simulink model "BenchmarkModel_Dynamic_TestCase"  (R2020a)
settings: Solver=ode45  StartTime=0.0  StopTime=5  RelTol=1e-3
undefined symbols (not defined in the file): Angle, D1, Delta, find_system, Magnitude
libraries: powerlib x91, powerlib_meascontrol x31, simulink x6, dspsrcs4 x3, dspsigops x2, sps_avr x1
(part 1 of 3)
settings Model: Creator=user  LastModifiedBy=anton

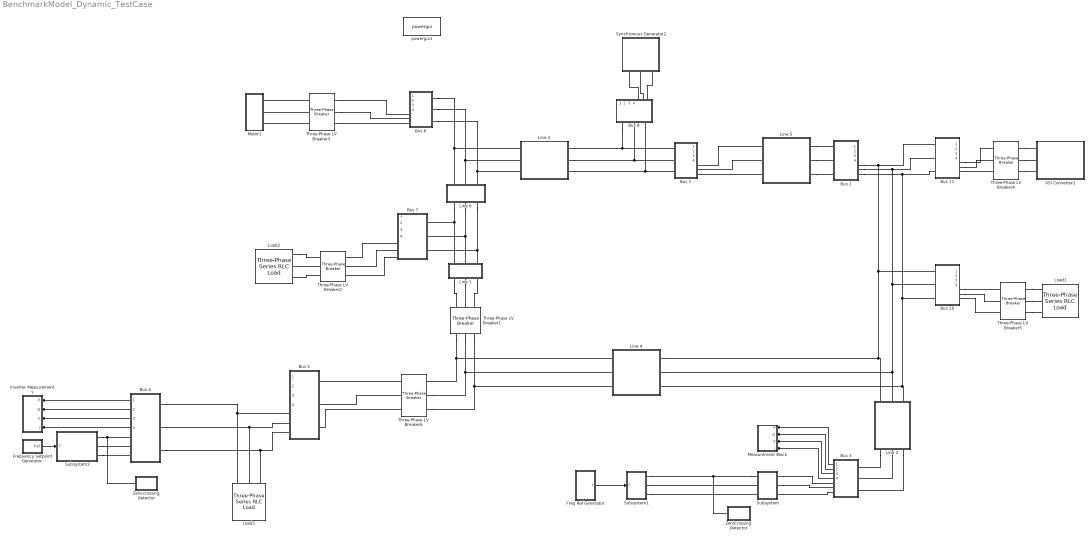
== system BenchmarkModel_Dynamic_TestCase ==
  Bus {1..8,10..11} (10 alike) : Subsystem  ReferencedSubsystem=Bus
  Freq Ref Generator : Subsystem
  Frequency Setpoint Generator : Subsystem
  Inverter Measurements : Subsystem
  Line 1 : Subsystem  mask{Rline=0.497*3, Lline=0.086*3/(2*pi*50)}
      mask prompts: Rline "Resistance"; Lline "Reactance"
      mask DialogControl DescTextVar Prompt: Line block for LV grid
  Line 2 : Subsystem  mask{Rline=0.497*0.5, Lline=0.086*0.5/(2*pi*50)}
      mask prompts: Rline "Resistance"; Lline "Reactance"
      mask DialogControl DescTextVar Prompt: Line block for LV grid
  Line 3 : Subsystem  mask{Rline=0.497*0.5, Lline=0.086*0.5/(2*pi*50)}
      mask prompts: Rline "Resistance"; Lline "Reactance"
      mask DialogControl DescTextVar Prompt: Line block for LV grid
  Line 4 : Subsystem  mask{Rline=0.497*3, Lline=0.086*3/(2*pi*50)}
      mask prompts: Rline "Resistance"; Lline "Reactance"
      mask DialogControl DescTextVar Prompt: Line block for LV grid
  Line 5 : Subsystem  mask{Rline=0.497, Lline=0.086/(2*pi*50)}
      mask prompts: Rline "Resistance"; Lline "Reactance"
      mask DialogControl DescTextVar Prompt: Line block for LV grid
  Line 6 : Subsystem  mask{Rline=0.497*0.5, Lline=0.086*0.5/(2*pi*50)}
      mask prompts: Rline "Resistance"; Lline "Reactance"
      mask DialogControl DescTextVar Prompt: Line block for LV grid
  Load1 : powerlib/Elements/Three-Phase Series RLC Load  LConnTagsString=A|B|C  Configuration=Y (grounded)  NominalVoltage=420  Vabc=[1e3 1e3 1e3]  Vabcp=[1e3 1e3 1e3]  NominalFrequency=50  UnbalancedPower=off  ActivePower=10e3  InductivePower=1e3  CapacitivePower=0  Pabc=[10e3 9e3 11e3]  QLabc=[100 90 110]  QCabc=[100 90 110]  Pabcp=[10e3 9e3 11e3]  QLabcp=[100 90 110]  QCabcp=[100 90 110]  Measurements=None  LoadType=constant Z
  Load2 : powerlib/Elements/Three-Phase Series RLC Load  LConnTagsString=A|B|C  Configuration=Y (grounded)  NominalVoltage=420  Vabc=[1e3 1e3 1e3]  Vabcp=[1e3 1e3 1e3]  NominalFrequency=50  UnbalancedPower=off  ActivePower=10e3  InductivePower=1e3  CapacitivePower=0  Pabc=[10e3 9e3 11e3]  QLabc=[100 90 110]  QCabc=[100 90 110]  Pabcp=[10e3 9e3 11e3]  QLabcp=[100 90 110]  QCabcp=[100 90 110]  Measurements=None  LoadType=constant Z
  Load3 : powerlib/Elements/Three-Phase Series RLC Load  LConnTagsString=A|B|C  Configuration=Y (grounded)  NominalVoltage=420  Vabc=[1e3 1e3 1e3]  Vabcp=[1e3 1e3 1e3]  NominalFrequency=50  UnbalancedPower=off  ActivePower=2e3  InductivePower=0  CapacitivePower=0  Pabc=[10e3 9e3 11e3]  QLabc=[100 90 110]  QCabc=[100 90 110]  Pabcp=[10e3 9e3 11e3]  QLabcp=[100 90 110]  QCabcp=[100 90 110]  Measurements=None  LoadType=constant Z
  Measurement Block : Subsystem
  Motor1 : Subsystem
  Subsystem : Subsystem
  Subsystem1 : Subsystem
  Subsystem2 : Subsystem
  Synchronous Generator2 : Subsystem
  Three-Phase LV Breaker{1..5} (5 alike) : powerlib/Elements/Three-Phase Breaker  InitialState=closed  SwitchA=on  SwitchB=on  SwitchC=on  SwitchTimes=10  External=off  BreakerResistance=0.001  SnubberResistance=1e5  SnubberCapacitance=inf  Measurements=None
  Three-Phase LV Breaker6 : powerlib/Elements/Three-Phase Breaker  InitialState=closed  SwitchA=on  SwitchB=on  SwitchC=on  SwitchTimes=2  External=off  BreakerResistance=0.001  SnubberResistance=1e5  SnubberCapacitance=inf  Measurements=None
  VSI Converter1 : Subsystem  mask{Pmax=50000, Qmax=50000, Vdc=760, fsw=5000, L1t=640e-6, Lf=63e-6, Cf=100e-6}
      mask prompts: Pmax "Max Active Power [VAr]"; Qmax "Max Reactive Power [VAr]"; Vdc "DC bus Voltage [V]"; fsw "Switching Frequency [Hz]"; L1t "Filter Inductance [H]"; Lf "Output Inductance [H]"; Cf "Filter Capacitance [F]"
      mask Display: disp(' ');
  Zero-crossing detector : Subsystem
  ZeroCrossing Detector : Subsystem
  powergui1 : powerlib/powergui  Priority=1  SimulationMode=Discrete  SampleTime=5e-6  frequency=50  Iterations=50  frequencyindice=0  Pbase=100e6  ErrMax=1e-4  UnitsV=kV  UnitsW=MW  buscounter=0  FunctionMessages=off  echomessages=off  EnableUseOfTLC=off  CurrentSourceSwitches=off  DisableSnubberDevices=off  DisableRonSwitches=off  DisableVfSwitches=off  DisplayEquations=off  AutomaticDiscreteSolvers=off  SolverType=Tustin/Backward Euler (TBE)  Interpol=off  ExternalGateDelay=off  methode=off  Ts=100  x0status=blocks  SPID=on  SwTol=0  HookPort=off  NonlinearTolerance=1e-4  nMaxIteration=100  ContinueOnMaxIteration=off  RestoreLinks=warning  ResistiveCurrentMeasurement=off  Frange=[0:2:500]  Ylog=off  Xlog=on  ShowGrid=off  save=off  variable=ZData  structure=0  ZoomFFT=off  StartTime=0.0  cycles=1  DisplayStyle=1  fundamental=60  FreqAxis=off  MaxFrequency=1000  frequencyindicesteady=1  RmsSteady=1  display=off
  wires:
  Bus 4/1 -> Inverter Measurements/1(P)
  Bus 4/2 -> Inverter Measurements/2(Q)
  Bus 4/3 -> Inverter Measurements/3(V)
  Bus 4/4 -> Inverter Measurements/4(I)
  Frequency Setpoint Generator/1(fref) -> Subsystem2/1(f)
  Freq Ref Generator/1(f) -> Subsystem1/1(f)
  Bus 3/1 -> Measurement Block/1(P)
  Bus 3/2 -> Measurement Block/2(Q)
  Bus 3/3 -> Measurement Block/3(V)
  Bus 3/4 -> Measurement Block/4(I)
  connections:
  Bus 10/LConn2 -- Bus 11/LConn2 -- Bus 2/RConn2 -- Line 4/LConn2 -- Line 2/LConn2
  Bus 10/LConn3 -- Bus 11/LConn3 -- Bus 2/RConn3 -- Line 4/LConn3 -- Line 2/LConn3
  Subsystem/RConn3 -- Bus 3/RConn3
  Subsystem/RConn2 -- Bus 3/RConn2
  Subsystem/RConn1 -- Bus 3/RConn1
  Line 2/RConn1 -- Bus 3/LConn1
  Line 2/RConn2 -- Bus 3/LConn2
  Line 2/RConn3 -- Bus 3/LConn3
  Line 5/RConn3 -- Bus 1/RConn3
  Line 5/RConn2 -- Bus 1/RConn2
  Line 5/RConn1 -- Bus 1/RConn1
  Line 5/LConn3 -- Bus 2/LConn3
  Line 5/LConn2 -- Bus 2/LConn2
  Line 5/LConn1 -- Bus 2/LConn1
  Bus 6/LConn3 -- Line 3/RConn3 -- Line 6/LConn3
  Bus 1/LConn2 -- Line 3/LConn2 -- Bus 8/LConn2
  Bus 6/LConn1 -- Line 6/LConn1 -- Line 3/RConn1
  Line 1/RConn2 -- Three-Phase LV Breaker1/RConn2
  Line 1/RConn1 -- Three-Phase LV Breaker1/RConn1
  Line 1/RConn3 -- Three-Phase LV Breaker1/RConn3
  Bus 2/RConn1 -- Line 2/LConn1 -- Line 4/LConn1 -- Bus 10/LConn1 -- Bus 11/LConn1
  Three-Phase LV Breaker1/LConn2 -- Three-Phase LV Breaker6/RConn2 -- Line 4/RConn2
  Three-Phase LV Breaker1/LConn1 -- Three-Phase LV Breaker6/RConn1 -- Line 4/RConn1
  Three-Phase LV Breaker1/LConn3 -- Three-Phase LV Breaker6/RConn3 -- Line 4/RConn3
  Bus 8/RConn1 -- Synchronous Generator2/RConn1
  Bus 8/RConn2 -- Synchronous Generator2/RConn2
  Bus 8/RConn3 -- Synchronous Generator2/RConn3
  Load2/LConn1 -- Three-Phase LV Breaker2/LConn1
  Load2/LConn2 -- Three-Phase LV Breaker2/LConn2
  Load2/LConn3 -- Three-Phase LV Breaker2/LConn3
  Bus 7/RConn1 -- Three-Phase LV Breaker2/RConn1
  Bus 7/RConn2 -- Three-Phase LV Breaker2/RConn2
  Bus 7/RConn3 -- Three-Phase LV Breaker2/RConn3
  Three-Phase LV Breaker3/LConn1 -- Motor1/LConn1
  Three-Phase LV Breaker3/LConn2 -- Motor1/LConn2
  Three-Phase LV Breaker3/LConn3 -- Motor1/LConn3
  Three-Phase LV Breaker3/RConn3 -- Bus 6/RConn3
  Three-Phase LV Breaker3/RConn2 -- Bus 6/RConn2
  Three-Phase LV Breaker3/RConn1 -- Bus 6/RConn1
  Three-Phase LV Breaker4/LConn1 -- VSI Converter1/LConn1
  Three-Phase LV Breaker4/LConn2 -- VSI Converter1/LConn2
  Three-Phase LV Breaker4/LConn3 -- VSI Converter1/LConn3
  Bus 11/RConn1 -- Three-Phase LV Breaker4/RConn1
  Bus 11/RConn2 -- Three-Phase LV Breaker4/RConn2
  Bus 11/RConn3 -- Three-Phase LV Breaker4/RConn3
  Three-Phase LV Breaker5/LConn1 -- Load1/LConn1
  Three-Phase LV Breaker5/LConn2 -- Load1/LConn2
  Three-Phase LV Breaker5/LConn3 -- Load1/LConn3
  Bus 10/RConn1 -- Three-Phase LV Breaker5/RConn1
  Bus 10/RConn2 -- Three-Phase LV Breaker5/RConn2
  Bus 10/RConn3 -- Three-Phase LV Breaker5/RConn3
  Bus 5/RConn1 -- Bus 4/LConn1 -- Load3/LConn1
  Bus 5/RConn2 -- Bus 4/LConn2 -- Load3/LConn2
  Bus 5/RConn3 -- Bus 4/LConn3 -- Load3/LConn3
  Subsystem1/RConn2 -- Subsystem/LConn2
  Subsystem1/RConn3 -- Subsystem/LConn3
  Bus 5/LConn1 -- Three-Phase LV Breaker6/LConn1
  Bus 5/LConn2 -- Three-Phase LV Breaker6/LConn2
  Bus 5/LConn3 -- Three-Phase LV Breaker6/LConn3
  Subsystem2/RConn1 -- Zero-crossing detector/LConn1 -- Bus 4/RConn1
  Subsystem2/RConn2 -- Bus 4/RConn2
  Subsystem2/RConn3 -- Bus 4/RConn3
  Bus 1/LConn3 -- Line 3/LConn3 -- Bus 8/LConn3
  Bus 8/LConn1 -- Line 3/LConn1 -- Bus 1/LConn1
  Bus 6/LConn2 -- Line 6/LConn2 -- Line 3/RConn2
  Line 1/LConn1 -- Line 6/RConn1 -- Bus 7/LConn1
  Line 1/LConn2 -- Line 6/RConn2 -- Bus 7/LConn2
  Line 1/LConn3 -- Line 6/RConn3 -- Bus 7/LConn3
  Subsystem/LConn1 -- ZeroCrossing Detector/LConn1 -- Subsystem1/RConn1

== system BenchmarkModel_Dynamic_TestCase/Freq Ref Generator ==
  Constant : Constant  Value=50
  Ramp : simulink/Sources/Ramp  slope=0.5  start=2  InitialOutput=0
  Ramp1 : simulink/Sources/Ramp  slope=-0.5  start=1  InitialOutput=0
  Sum : Sum  Inputs=|+++
  f : Outport
  wires:
  Sum/1 -> f/1
  Constant/1 -> Sum/1
  Ramp1/1 -> Sum/3
  Ramp/1 -> Sum/2

== system BenchmarkModel_Dynamic_TestCase/Frequency Setpoint Generator ==
  Constant1 : Constant  Value=50
  Constant2 : Constant  Value=20
  Ground : Ground
  Switch : Switch  Criteria=u2 > Threshold  Threshold=10
  fref : Outport
  wires:
  Constant1/1 -> Switch/1
  Ground/1 -> Switch/3
  Constant2/1 -> Switch/2
  Switch/1 -> fref/1

== system BenchmarkModel_Dynamic_TestCase/Inverter Measurements ==
  P : Inport
  Q : Inport  Port=2
  V : Inport  Port=3
  I : Inport  Port=4
  RMS : powerlib_meascontrol/Measurements/RMS  TrueRMS=on  Freq=50  RMSInit=220  Ts=0
  Signal conversion3 : Subsystem
  To Workspace : ToWorkspace  VariableName=PInverter  SaveFormat=Timeseries  SampleTime=-1
  To Workspace1 : ToWorkspace  VariableName=QInverter  SaveFormat=Timeseries  SampleTime=-1
  To Workspace2 : ToWorkspace  VariableName=VdInverter  SaveFormat=Timeseries  SampleTime=-1
  To Workspace3 : ToWorkspace  VariableName=Vqinverter  SaveFormat=Timeseries  SampleTime=-1
  To Workspace6 : ToWorkspace  VariableName=IdInverter  SaveFormat=Timeseries  SampleTime=-1
  To Workspace7 : ToWorkspace  VariableName=IqInverter  SaveFormat=Timeseries  SampleTime=-1
  To Workspace8 : ToWorkspace  VariableName=VInverter  SaveFormat=Timeseries  SampleTime=-1
  To Workspace9 : ToWorkspace  VariableName=VRMSInverter  SaveFormat=Timeseries  SampleTime=-1
  wires:
  Signal conversion3/1(Vd) -> To Workspace2/1
  V/1 -> To Workspace8/1, RMS/1, Signal conversion3/1(Vsabc)
  P/1 -> To Workspace/1
  Signal conversion3/2(Vq) -> To Workspace3/1
  Signal conversion3/3(ILd) -> To Workspace6/1
  I/1 -> Signal conversion3/2(ILabc)
  Signal conversion3/4(ILq) -> To Workspace7/1
  RMS/1 -> To Workspace9/1
  Q/1 -> To Workspace1/1

== system BenchmarkModel_Dynamic_TestCase/Line 1 ==
  Series RLC BranchA : powerlib/Elements/Series RLC Branch  LConnTagsString=__new0  RConnTagsString=__new0  BranchType=RL  Resistance=Rline  Inductance=Lline  SetiL0=off  InitialCurrent=0  Capacitance=1e-6  Setx0=off  InitialVoltage=0  Measurements=None
  Series RLC BranchB : powerlib/Elements/Series RLC Branch  LConnTagsString=__new0  RConnTagsString=__new0  BranchType=RL  Resistance=Rline  Inductance=Lline  SetiL0=off  InitialCurrent=0  Capacitance=1e-6  Setx0=off  InitialVoltage=0  Measurements=None
  Series RLC BranchC : powerlib/Elements/Series RLC Branch  LConnTagsString=__new0  RConnTagsString=__new0  BranchType=RL  Resistance=Rline  Inductance=Lline  SetiL0=off  InitialCurrent=0  Capacitance=1e-6  Setx0=off  InitialVoltage=0  Measurements=None
  a : PMIOPort  Side=Left
  A : PMIOPort  Port=2  Side=Right
  b : PMIOPort  Port=3  Side=Left
  B : PMIOPort  Port=4  Side=Right
  c : PMIOPort  Port=5  Side=Left
  C : PMIOPort  Port=6  Side=Right
  connections:
  Series RLC BranchB/RConn1 -- B/RConn1
  Series RLC BranchC/RConn1 -- C/RConn1
  Series RLC BranchB/LConn1 -- b/RConn1
  Series RLC BranchA/RConn1 -- A/RConn1
  Series RLC BranchA/LConn1 -- a/RConn1
  Series RLC BranchC/LConn1 -- c/RConn1

== system BenchmarkModel_Dynamic_TestCase/Line 2 ==
  Series RLC BranchA : powerlib/Elements/Series RLC Branch  LConnTagsString=__new0  RConnTagsString=__new0  BranchType=RL  Resistance=Rline  Inductance=Lline  SetiL0=off  InitialCurrent=0  Capacitance=1e-6  Setx0=off  InitialVoltage=0  Measurements=None
  Series RLC BranchB : powerlib/Elements/Series RLC Branch  LConnTagsString=__new0  RConnTagsString=__new0  BranchType=RL  Resistance=Rline  Inductance=Lline  SetiL0=off  InitialCurrent=0  Capacitance=1e-6  Setx0=off  InitialVoltage=0  Measurements=None
  Series RLC BranchC : powerlib/Elements/Series RLC Branch  LConnTagsString=__new0  RConnTagsString=__new0  BranchType=RL  Resistance=Rline  Inductance=Lline  SetiL0=off  InitialCurrent=0  Capacitance=1e-6  Setx0=off  InitialVoltage=0  Measurements=None
  a : PMIOPort  Side=Left
  A : PMIOPort  Port=2  Side=Right
  b : PMIOPort  Port=3  Side=Left
  B : PMIOPort  Port=4  Side=Right
  c : PMIOPort  Port=5  Side=Left
  C : PMIOPort  Port=6  Side=Right
  connections:
  Series RLC BranchC/LConn1 -- c/RConn1
  Series RLC BranchA/LConn1 -- a/RConn1
  Series RLC BranchA/RConn1 -- A/RConn1
  Series RLC BranchB/LConn1 -- b/RConn1
  Series RLC BranchC/RConn1 -- C/RConn1
  Series RLC BranchB/RConn1 -- B/RConn1

== system BenchmarkModel_Dynamic_TestCase/Line 3 ==
  Series RLC BranchA : powerlib/Elements/Series RLC Branch  LConnTagsString=__new0  RConnTagsString=__new0  BranchType=RL  Resistance=Rline  Inductance=Lline  SetiL0=off  InitialCurrent=0  Capacitance=1e-6  Setx0=off  InitialVoltage=0  Measurements=None
  Series RLC BranchB : powerlib/Elements/Series RLC Branch  LConnTagsString=__new0  RConnTagsString=__new0  BranchType=RL  Resistance=Rline  Inductance=Lline  SetiL0=off  InitialCurrent=0  Capacitance=1e-6  Setx0=off  InitialVoltage=0  Measurements=None
  Series RLC BranchC : powerlib/Elements/Series RLC Branch  LConnTagsString=__new0  RConnTagsString=__new0  BranchType=RL  Resistance=Rline  Inductance=Lline  SetiL0=off  InitialCurrent=0  Capacitance=1e-6  Setx0=off  InitialVoltage=0  Measurements=None
  a : PMIOPort  Side=Left
  A : PMIOPort  Port=2  Side=Right
  b : PMIOPort  Port=3  Side=Left
  B : PMIOPort  Port=4  Side=Right
  c : PMIOPort  Port=5  Side=Left
  C : PMIOPort  Port=6  Side=Right
  connections:
  Series RLC BranchB/RConn1 -- B/RConn1
  Series RLC BranchC/RConn1 -- C/RConn1
  Series RLC BranchB/LConn1 -- b/RConn1
  Series RLC BranchA/RConn1 -- A/RConn1
  Series RLC BranchA/LConn1 -- a/RConn1
  Series RLC BranchC/LConn1 -- c/RConn1

== system BenchmarkModel_Dynamic_TestCase/Line 4 ==
  Series RLC BranchA : powerlib/Elements/Series RLC Branch  LConnTagsString=__new0  RConnTagsString=__new0  BranchType=RL  Resistance=Rline  Inductance=Lline  SetiL0=off  InitialCurrent=0  Capacitance=1e-6  Setx0=off  InitialVoltage=0  Measurements=None
  Series RLC BranchB : powerlib/Elements/Series RLC Branch  LConnTagsString=__new0  RConnTagsString=__new0  BranchType=RL  Resistance=Rline  Inductance=Lline  SetiL0=off  InitialCurrent=0  Capacitance=1e-6  Setx0=off  InitialVoltage=0  Measurements=None
  Series RLC BranchC : powerlib/Elements/Series RLC Branch  LConnTagsString=__new0  RConnTagsString=__new0  BranchType=RL  Resistance=Rline  Inductance=Lline  SetiL0=off  InitialCurrent=0  Capacitance=1e-6  Setx0=off  InitialVoltage=0  Measurements=None
  a : PMIOPort  Side=Left
  A : PMIOPort  Port=2  Side=Right
  b : PMIOPort  Port=3  Side=Left
  B : PMIOPort  Port=4  Side=Right
  c : PMIOPort  Port=5  Side=Left
  C : PMIOPort  Port=6  Side=Right
  connections:
  Series RLC BranchB/RConn1 -- B/RConn1
  Series RLC BranchC/RConn1 -- C/RConn1
  Series RLC BranchB/LConn1 -- b/RConn1
  Series RLC BranchA/RConn1 -- A/RConn1
  Series RLC BranchA/LConn1 -- a/RConn1
  Series RLC BranchC/LConn1 -- c/RConn1

== system BenchmarkModel_Dynamic_TestCase/Line 5 ==
  Series RLC BranchA : powerlib/Elements/Series RLC Branch  LConnTagsString=__new0  RConnTagsString=__new0  BranchType=RL  Resistance=Rline  Inductance=Lline  SetiL0=off  InitialCurrent=0  Capacitance=1e-6  Setx0=off  InitialVoltage=0  Measurements=None
  Series RLC BranchB : powerlib/Elements/Series RLC Branch  LConnTagsString=__new0  RConnTagsString=__new0  BranchType=RL  Resistance=Rline  Inductance=Lline  SetiL0=off  InitialCurrent=0  Capacitance=1e-6  Setx0=off  InitialVoltage=0  Measurements=None
  Series RLC BranchC : powerlib/Elements/Series RLC Branch  LConnTagsString=__new0  RConnTagsString=__new0  BranchType=RL  Resistance=Rline  Inductance=Lline  SetiL0=off  InitialCurrent=0  Capacitance=1e-6  Setx0=off  InitialVoltage=0  Measurements=None
  a : PMIOPort  Side=Left
  A : PMIOPort  Port=2  Side=Right
  b : PMIOPort  Port=3  Side=Left
  B : PMIOPort  Port=4  Side=Right
  c : PMIOPort  Port=5  Side=Left
  C : PMIOPort  Port=6  Side=Right
  connections:
  Series RLC BranchB/RConn1 -- B/RConn1
  Series RLC BranchC/RConn1 -- C/RConn1
  Series RLC BranchB/LConn1 -- b/RConn1
  Series RLC BranchA/RConn1 -- A/RConn1
  Series RLC BranchA/LConn1 -- a/RConn1
  Series RLC BranchC/LConn1 -- c/RConn1

== system BenchmarkModel_Dynamic_TestCase/Line 6 ==
  Series RLC BranchA : powerlib/Elements/Series RLC Branch  LConnTagsString=__new0  RConnTagsString=__new0  BranchType=RL  Resistance=Rline  Inductance=Lline  SetiL0=off  InitialCurrent=0  Capacitance=1e-6  Setx0=off  InitialVoltage=0  Measurements=None
  Series RLC BranchB : powerlib/Elements/Series RLC Branch  LConnTagsString=__new0  RConnTagsString=__new0  BranchType=RL  Resistance=Rline  Inductance=Lline  SetiL0=off  InitialCurrent=0  Capacitance=1e-6  Setx0=off  InitialVoltage=0  Measurements=None
  Series RLC BranchC : powerlib/Elements/Series RLC Branch  LConnTagsString=__new0  RConnTagsString=__new0  BranchType=RL  Resistance=Rline  Inductance=Lline  SetiL0=off  InitialCurrent=0  Capacitance=1e-6  Setx0=off  InitialVoltage=0  Measurements=None
  a : PMIOPort  Side=Left
  A : PMIOPort  Port=2  Side=Right
  b : PMIOPort  Port=3  Side=Left
  B : PMIOPort  Port=4  Side=Right
  c : PMIOPort  Port=5  Side=Left
  C : PMIOPort  Port=6  Side=Right
  connections:
  Series RLC BranchB/RConn1 -- B/RConn1
  Series RLC BranchC/RConn1 -- C/RConn1
  Series RLC BranchB/LConn1 -- b/RConn1
  Series RLC BranchA/RConn1 -- A/RConn1
  Series RLC BranchA/LConn1 -- a/RConn1
  Series RLC BranchC/LConn1 -- c/RConn1

== system BenchmarkModel_Dynamic_TestCase/Measurement Block ==
  P : Inport
  Q : Inport  Port=2
  V : Inport  Port=3
  I : Inport  Port=4
  RMS1 : powerlib_meascontrol/Measurements/RMS  TrueRMS=on  Freq=50  RMSInit=220  Ts=0
  Signal conversion2 : Subsystem
  To Workspace10 : ToWorkspace  VariableName=VdGrid  SaveFormat=Timeseries  SampleTime=-1
  To Workspace11 : ToWorkspace  VariableName=VqGrid  SaveFormat=Timeseries  SampleTime=-1
  To Workspace12 : ToWorkspace  VariableName=IdGrid  SaveFormat=Timeseries  SampleTime=-1
  To Workspace13 : ToWorkspace  VariableName=IqGrid  SaveFormat=Timeseries  SampleTime=-1
  To Workspace14 : ToWorkspace  VariableName=PGrid  SaveFormat=Timeseries  SampleTime=-1
  To Workspace16 : ToWorkspace  VariableName=VGrid  SaveFormat=Timeseries  SampleTime=-1
  To Workspace17 : ToWorkspace  VariableName=VRMSGrid  SaveFormat=Timeseries  SampleTime=-1
  To Workspace18 : ToWorkspace  VariableName=QGrid  SaveFormat=Timeseries  SampleTime=-1
  wires:
  V/1 -> RMS1/1, To Workspace16/1, Signal conversion2/1(Vsabc)
  Signal conversion2/3(ILd) -> To Workspace12/1
  Signal conversion2/4(ILq) -> To Workspace13/1
  P/1 -> To Workspace14/1
  Q/1 -> To Workspace18/1
  Signal conversion2/1(Vd) -> To Workspace10/1
  I/1 -> Signal conversion2/2(ILabc)
  RMS1/1 -> To Workspace17/1
  Signal conversion2/2(Vq) -> To Workspace11/1

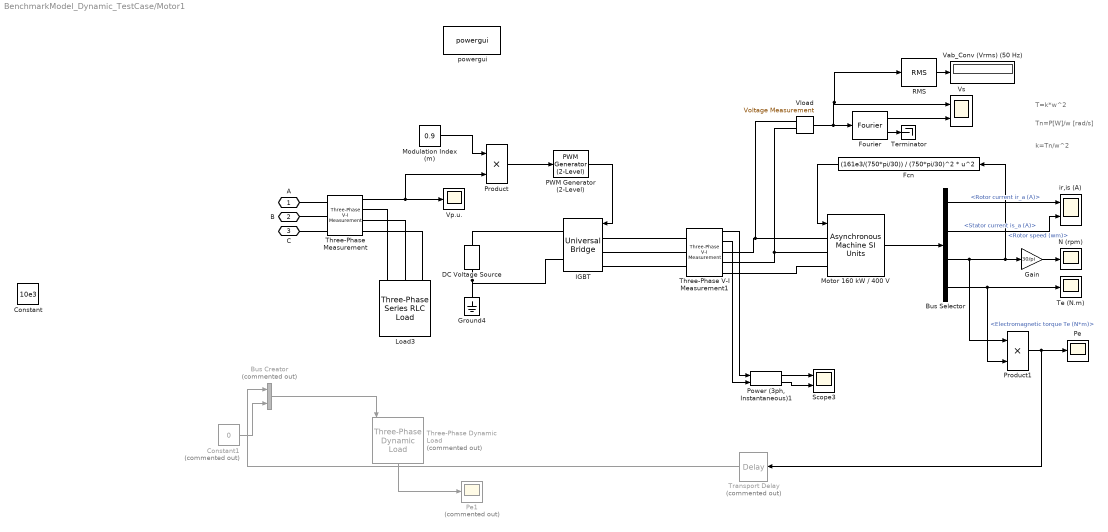
== system BenchmarkModel_Dynamic_TestCase/Motor1 ==
  note: Tn=P[W]/w [rad/s]
  note: k=Tn/w^2
  note: T=k*w^2
  Bus Creator : BusCreator  Commented=on  Inputs=2
  Bus Selector : BusSelector  OutputSignals=Rotor measurements.Rotor current ir_a (A),Stator measurements.Stator current is_a (A),Mechanical.Rotor speed (wm),Mechanical.Electromagnetic torque Te (N*m)
  Constant : Constant  Value=10e3
  Constant1 : Constant  Commented=on  Value=0
  DC Voltage Source : powerlib/Electrical Sources/DC Voltage Source  Amplitude=725  Measurements=None
  Fcn : Fcn  Expr=(161e3/(750*pi/30)) / (750*pi/30)^2 * u^2
  Fourier : powerlib_meascontrol/Measurements/Fourier  Freq=50  n=1  InInit=[0, 0]  Ts=10e-6
  Gain : Gain  Gain=30/pi
  Ground4 : powerlib/Elements/Ground  LConnTagsString=a
  IGBT : powerlib/Power Electronics/Universal Bridge  Arms=3  SnubberResistance=1e5  SnubberCapacitance=inf  Device=IGBT / Diodes  Ron=1e-3  Lon=0  ForwardVoltages="[  0  0  ]"  ForwardVoltage=0  GTOparameters=[ 10e-6 , 20e-6 ]  IGBTparameters=[ 1e-6 , 2e-6 ]  Measurements=None  Measurements_2=None  converterType=Rectifier
  Load3 : powerlib/Elements/Three-Phase Series RLC Load  LConnTagsString=A|B|C  Configuration=Y (grounded)  NominalVoltage=400  Vabc=[1e3 1e3 1e3]  Vabcp=[1e3 1e3 1e3]  NominalFrequency=50  UnbalancedPower=off  ActivePower=10e3  InductivePower=0  CapacitivePower=0  Pabc=[10e3 9e3 11e3]  QLabc=[100 90 110]  QCabc=[100 90 110]  Pabcp=[10e3 9e3 11e3]  QLabcp=[100 90 110]  QCabcp=[100 90 110]  Measurements=None  LoadType=constant Z
  Modulation Index (m) : Constant  Value=0.9  SampleTime=10e-6
  Motor 160 kW / 400 V : powerlib/Machines/Asynchronous Machine SI Units  RotorType=Squirrel-cage  PresetModel=No  MechanicalLoad=Torque Tm  ShowDetailedParameters=on  ReferenceFrame=Rotor  Units=SI  MeasurementBus=off  NominalParameters=[1.6e+05 400 50]  Stator=[0.01379 0.000152]  Rotor=[0.007728 0.000152]  Cage1=[0.01779 0.0006371]  Cage2=[0.05053 0.0002281]  Lm=0.00769  Mechanical=[2.9 0.05658 2]  PolePairs=2  InitialConditions=[1 0 0 0 0 0 -120 120]  SimulateSaturation=off  Saturation=[14.03593122, 27.81365428, 53.79336849, 72.68890987, 97.98006896, 148.6815601, 215.7428561, 302.9841135, 420.4778367 ; 230, 322, 414, 460, 506, 552, 598, 644, 690]  LoadFlowParameters=200000  TsPowergui=0  TsBlock=-1  IterativeModel=Trapezoidal non iterative  IterativeDiscreteModel=Trapezoidal non iterative  Pmec=0
  N (rpm) : Scope
  PWM Generator (2-Level) : powerlib_meascontrol/Pulse & Signal Generators/PWM Generator (2-Level)  ModulatorType=Three-phase bridge (6 pulses)  ModulatorMode=Unsynchronized  Fc=33*50  Pc=0  nF=27  MinMax="[ -1  1 ]"  SamplingTechnique=Natural  ModulatingSignals=off  m=0.9  Freq=50  Phase=0  Ts=10e-6  ShowCarrierOutport=off
  Pe : Scope
  Pe1 : Scope  Commented=on
  "Power (3ph, Instantaneous)1" : powerlib_meascontrol/Measurements/Power (3ph, Instantaneous)
  Product : Product  RndMeth=Zero  SampleTime=10e-6
  Product1 : Product  RndMeth=Zero  SampleTime=10e-6
  RMS : powerlib_meascontrol/Measurements/RMS  TrueRMS=off  Freq=50  RMSInit=400  Ts=10e-6
  Scope3 : Scope  NumInputPorts=2
  Te (N.m) : Scope
  Terminator : Terminator
  Three-Phase Dynamic Load : powerlib/Elements/Three-Phase Dynamic Load  Commented=on  NominalVoltage=[ 400 50 ]  ActiveReactivePowers=[0 0]  PositiveSequence=[0.994 -11.8]  ExternalControl=on  NpNq=[1.3 2]  TimeConstants="[0  0  0  0]"  MinimumVoltage=0.7  Tfilter=1e-4  LoadFlowParameters=[4,0,0,0,0]
      settings: SourceProductBaseCode=PS
  Three-Phase Measurement : powerlib/Measurements/Three-Phase V-I Measurement  VoltageMeasurement=phase-to-ground  SetLabelV=off  LabelV=Vabc  Vpu=on  VpuLL=off  CurrentMeasurement=no  SetLabelI=off  LabelI=Iabc  Ipu=off  Pbase=100e6  Vbase=420  OutputType=Complex  PhasorSimulation=off  PSBequivalent=0
  Three-Phase V-I Measurement1 : powerlib/Measurements/Three-Phase V-I Measurement  VoltageMeasurement=phase-to-ground  SetLabelV=off  LabelV=Vabc  Vpu=off  VpuLL=off  CurrentMeasurement=yes  SetLabelI=off  LabelI=Iabc  Ipu=off  Pbase=100e6  Vbase=500e3  OutputType=Complex  PhasorSimulation=off  PSBequivalent=0
  Transport Delay : TransportDelay  Commented=on  DelayTime=0.01
  Vab_Conv (Vrms) (50 Hz) : Display
      settings: Decimation=100
  Vload : powerlib/Measurements/Voltage Measurement  Tag=PoWeRsYsTeMmEaSuReMeNt  PhasorSimulation=off  OutputType=Magnitude  PSBequivalent=0
  Vp.u. : Scope
  Vs : Scope  NumInputPorts=2
  ir,is (A) : Scope  NumInputPorts=2
  powergui : powerlib/powergui  Priority=1  SimulationMode=Discrete  SampleTime=10e-6  frequency=50  Iterations=50  frequencyindice=50  Pbase=100e6  ErrMax=0.0001  UnitsV=kV  UnitsW=MW  buscounter=0  FunctionMessages=off  echomessages=off  EnableUseOfTLC=off  CurrentSourceSwitches=off  DisableSnubberDevices=off  DisableRonSwitches=off  DisableVfSwitches=off  DisplayEquations=off  AutomaticDiscreteSolvers=off  SolverType=Tustin/Backward Euler (TBE)  Interpol=off  ExternalGateDelay=off  methode=off  Ts=100  x0status=blocks  SPID=on  SwTol=0  HookPort=off  NonlinearTolerance=1e-4  nMaxIteration=100  ContinueOnMaxIteration=off  RestoreLinks=warning  ResistiveCurrentMeasurement=off  Frange=[0:2:500]  Ylog=off  Xlog=on  ShowGrid=off  save=off  variable=ZData  structure=0  ZoomFFT=off  StartTime=0.0  cycles=1  DisplayStyle=1  fundamental=60  FreqAxis=off  MaxFrequency=1000  frequencyindicesteady=1  RmsSteady=1  display=off
  A : PMIOPort  Side=Left
  B : PMIOPort  Port=2  Side=Left
  C : PMIOPort  Port=3  Side=Left
  wires:
  Bus Selector/2 -> ir,is (A)/2  "<Stator current is_a (A)>"
  RMS/1 -> Vab_Conv (Vrms) (50 Hz)/1
  Modulation Index (m)/1 -> Product/1
  Three-Phase Measurement/1 -> Vp.u./1, Product/2
  Fcn/1 -> Motor 160 kW / 400 V/1
  Fourier/2 -> Terminator/1
  Fourier/1 -> Vs/2
  Bus Selector/3 -> Product1/1, Gain/1, Fcn/1  "<Rotor speed (wm)>"
  Product/1 -> PWM Generator (2-Level)/1
  Motor 160 kW / 400 V/1 -> Bus Selector/1
  Bus Selector/4 -> Product1/2, Te (N.m)/1  "<Electromagnetic torque Te (N*m)>"
  PWM Generator (2-Level)/1 -> IGBT/1
  Bus Selector/1 -> ir,is (A)/1  "<Rotor current ir_a (A)>"
  Vload/1 -> Fourier/1, RMS/1, Vs/1
  Gain/1 -> N (rpm)/1
  Bus Creator/1 -> Three-Phase Dynamic Load/1
  Product1/1 -> Transport Delay/1, Pe/1
  Constant1/1 -> Bus Creator/2
  Three-Phase V-I Measurement1/2 -> "Power (3ph, Instantaneous)1"/2
  Three-Phase V-I Measurement1/1 -> "Power (3ph, Instantaneous)1"/1
  "Power (3ph, Instantaneous)1"/1 -> Scope3/1
  "Power (3ph, Instantaneous)1"/2 -> Scope3/2
  Three-Phase Dynamic Load/1 -> Pe1/1
  Transport Delay/1 -> Bus Creator/1
  connections:
  Three-Phase Measurement/LConn3 -- C/RConn1
  Three-Phase Measurement/LConn1 -- A/RConn1
  Three-Phase Measurement/LConn2 -- B/RConn1
  DC Voltage Source/LConn1 -- Ground4/LConn1 -- IGBT/RConn2
  DC Voltage Source/RConn1 -- IGBT/RConn1
  IGBT/LConn1 -- Three-Phase V-I Measurement1/LConn1
  IGBT/LConn2 -- Three-Phase V-I Measurement1/LConn2
  IGBT/LConn3 -- Three-Phase V-I Measurement1/LConn3
  Three-Phase V-I Measurement1/RConn3 -- Motor 160 kW / 400 V/LConn3
  Three-Phase V-I Measurement1/RConn2 -- Vload/LConn2 -- Motor 160 kW / 400 V/LConn2
  Three-Phase V-I Measurement1/RConn1 -- Vload/LConn1 -- Motor 160 kW / 400 V/LConn1
  Three-Phase Measurement/RConn1 -- Load3/LConn1
  Three-Phase Measurement/RConn2 -- Load3/LConn2
  Three-Phase Measurement/RConn3 -- Load3/LConn3

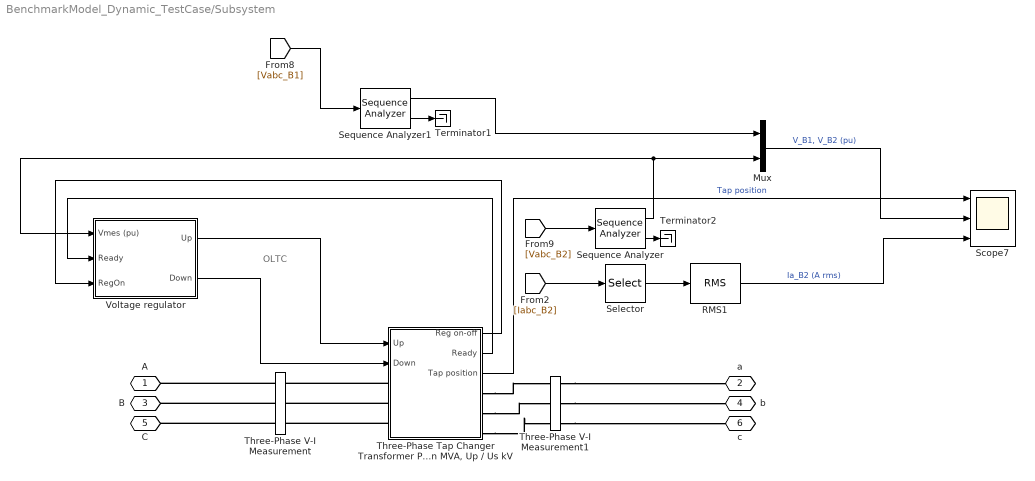
== system BenchmarkModel_Dynamic_TestCase/Subsystem ==
  note: OLTC
  Mux : Mux  Inputs=2
  RMS1 : powerlib_meascontrol/Measurements/RMS  TrueRMS=on  Freq=50  RMSInit=0  Ts=50e-6
  Scope7 : Scope  NumInputPorts=3
  Selector : Selector  InputPortWidth=3  IndexOptions=Index vector (dialog)  Indices=1  OutputSizes=1
  Sequence Analyzer : powerlib_meascontrol/Measurements/Sequence Analyzer  Freq=50  n=1  seq=Positive  InInit=[1, 0]  Ts=50e-6
      settings: SourceProductBaseCode=PS
  Sequence Analyzer1 : powerlib_meascontrol/Measurements/Sequence Analyzer  Freq=50  n=1  seq=Positive  InInit=[1, 0]  Ts=50e-6
      settings: SourceProductBaseCode=PS
  Terminator1 : Terminator
  Terminator2 : Terminator
  Three-Phase V-I Measurement : powerlib/Measurements/Three-Phase V-I Measurement  VoltageMeasurement=phase-to-ground  SetLabelV=on  LabelV=Vabc_B1  Vpu=on  VpuLL=off  CurrentMeasurement=no  SetLabelI=off  LabelI=Iabc  Ipu=off  Pbase=100e6  Vbase=20e3  OutputType=Complex  PhasorSimulation=off  PSBequivalent=0
  Three-Phase V-I Measurement1 : powerlib/Measurements/Three-Phase V-I Measurement  VoltageMeasurement=phase-to-ground  SetLabelV=on  LabelV=Vabc_B2  Vpu=on  VpuLL=off  CurrentMeasurement=yes  SetLabelI=on  LabelI=Iabc_B2  Ipu=off  Pbase=100e6  Vbase=0.42e3  OutputType=Complex  PhasorSimulation=off  PSBequivalent=0
  "Three-Phase Tap Changer Transformer Pn MVA, Up / Us kV" : Subsystem  LoadFcn=find_system(gcs,'FollowLinks', 'on', 'LookUnderMasks', 'all');  mask(Three-Phase OLTC Regulating Transformer Yg/D1){NominalParameters=[250e3 50], Winding1=[20e3 0.003 0.09], Winding2=[0.42e3 0.003 0.09], RXmag=[300 300], SetSaturation=off, SaturationCurrentFlux=[0 0; 0.002 1.0; 0.006 1.12; 0.009 1.15; 0.015 1.17; 0.03 1.19; 0.05 1.20; 0.08 1.21; 1.0 1.302], Flux_abc=[ -1.0 0.5 0.5], DeltaU=0.025, TapMinMax=[-4   4], InitialTap=0, TapSelectionTime=0.1, RegulatorOn=off, Regulator=[1.0  0.0375  0.4]}
      mask prompts: NominalParameters "Nominal power and frequency [ Pnom(VA)  Fnom(Hz)]:"; Winding1 "Winding 1 (Yg) [V2(Vrms Ph Ph) R1(pu)  X1(pu) ]:"; Winding2 "Winding 2 (D1) [V2(Vrms Ph Ph) R2(pu)  X2(pu) ]"; RXmag "Magnetization branch  [Rm(pu) Lm(pu)]"; SetSaturation "Simulate saturation:"; SaturationCurrentFlux "Saturation characteristic [i1 phi; i2 phi2; ....] (pu)"; Flux_abc "Initial fluxes  [ Flux_a  Flux_b  Flux_c ] (pu)"; DeltaU "Voltage step DeltaU per tap (pu)"; TapMinMax "Minimum and maximum tap positions"; InitialTap "Initial tap position"; TapSelectionTime "Tap selection time (s) (typical 3-10s)"; RegulatorOn "Voltage regulator"; Regulator "Voltage regulator [ Vref(pu) DeadBand(pu)  Delay(s)]"
      mask help:
      | Models a On Load Tap Changer (OLTC), three-phase , Yg-Delta transformer. The three-phase primary multi-tap winding is modeled with three Variable-Ratio Transformer blocks.
      |
      | The transformer voltage ratio U2/U1 (in pu) is given by:
      |                 U2/U1= 1/ (1+TapPosition*DeltaU)
      | Tap position 0 corresponds to nominal voltage ratio.
      |
      | In automatic mode, ('Voltage regulator'  'on'), the signal applied at the 'Vm' input is monitored and the voltage regulator asks for a tap change if:
      |                  abs(Vm-Vref)>DeadBand/2  during a time  t > Delay.
      mask init:
      | if InitialTap<TapMinMax(1) | InitialTap>TapMinMax(2)
      |    message = sprintf('The initial tap number must be an integer comprised between % d and %d',TapMinMax(1),TapMinMax(2));
      |    Erreur.message = message;
      |    Erreur.identifier = 'SimscapePowerSystemsST:OLTCTransformer:ParameterError';
      |    powericon('psberror',Erreur.message,Erreur.identifier,'NoUiwait');
      | end
      | 
      | Pnom=NominalParameters(1)/3;
      | Fnom=NominalParameters(2);
      | Vnom1= Winding1(1)/sqrt(3);
      | Vnom2=Winding2(1);
      | Rpu1= Winding1(2);
      | Rpu2=Winding2(2);
      | Xpu1= Winding1(3);
      | Xpu2=Winding2(3);
      | Rmpu=RXmag(1);
      | Lmpu=RXmag(2);
      | 
      | Zbase1=Vnom1^2/Pnom;
      | Zbase2=Vnom2^2/Pnom;
      | R1= Rpu1*Zbase1;
      | L1= Xpu1*Zbase1/(2*pi*Fnom);
      | R2= Rpu2*Zbase2;
      | L2= Xpu2*Zbase2/(2*pi*Fnom);
      | Rm=Rmpu*Zbase1;
      | Lm= Lmpu*Zbase1/(2*pi*Fnom);
      | 
      | % Saturation
      | if SetSaturation==1
      | 	set_param([gcb,'/Transformer_3Phase'],'SetSaturation','on');
      | else
      | 	set_param([gcb,'/Transformer_3Phase'],'SetSaturation','off');
      | end
      | 
      | RegulatorVref=Regulator(1);
      | RegulatorDeadBand=Regulator(2);
      | RegulatorDelay=Regulator(3);
      mask Callback SetSaturation:
      | tempMaskVis=get_param(gcb,'MaskVisibilities');
      | if strcmp(get_param(gcb,'SetSaturation'),'on')
      | 	tempMaskVis{6}='on';
      |     tempMaskVis{7}='on';
      | 	set_param(gcb,'MaskVisibilities',tempMaskVis);
      | else
      | 	tempMaskVis{6}='off';
      |     tempMaskVis{7}='off';
      | 	set_param(gcb,'MaskVisibilities',tempMaskVis);
      | end
      mask TypeOptions RegulatorOn: off | on
      mask Callback RegulatorOn:
      | tempMaskVis=get_param(gcb,'MaskVisibilities');
      | if strcmp(get_param(gcb,'RegulatorOn'),'on')
      | 	tempMaskVis{13}='on';
      | 	set_param(gcb,'MaskVisibilities',tempMaskVis);
      | else
      | 	tempMaskVis{13}='off';
      | 	set_param(gcb,'MaskVisibilities',tempMaskVis);
      | end
      mask DialogControl Container12 Prompt: Transformer
      mask DialogControl Container13 Prompt: OLTC and  Voltage Regulator
  Voltage regulator : Subsystem  mask{Vref=1.0, DeadBand=0.025, TimeDelay=0.1}
      mask prompts: Vref "Vref (pu)"; DeadBand "Deadband (pu)"; TimeDelay "Time delay (s)"
  A : PMIOPort  Side=Left
  a : PMIOPort  Port=2  Side=Right
  B : PMIOPort  Port=3  Side=Left
  b : PMIOPort  Port=4  Side=Right
  C : PMIOPort  Port=5  Side=Left
  c : PMIOPort  Port=6  Side=Right
  wires:
  Voltage regulator/2(Down) -> "Three-Phase Tap Changer Transformer Pn MVA, Up / Us kV"/2(Down)
  Mux/1 -> Scope7/2  "V_B1, V_B2 (pu)"
  Sequence Analyzer/2 -> Terminator2/1
  [Vabc_B2] -> Sequence Analyzer/1
  "Three-Phase Tap Changer Transformer Pn MVA, Up / Us kV"/2(Ready) -> Voltage regulator/2(Ready)
  Sequence Analyzer/1 -> Voltage regulator/1(Vmes (pu)), Mux/2
  RMS1/1 -> Scope7/3  "Ia_B2 (A rms)"
  Sequence Analyzer1/2 -> Terminator1/1
  Selector/1 -> RMS1/1
  Voltage regulator/1(Up) -> "Three-Phase Tap Changer Transformer Pn MVA, Up / Us kV"/1(Up)
  [Iabc_B2] -> Selector/1
  "Three-Phase Tap Changer Transformer Pn MVA, Up / Us kV"/1(Reg on-off) -> Voltage regulator/3(RegOn)
  [Vabc_B1] -> Sequence Analyzer1/1
  Sequence Analyzer1/1 -> Mux/1
  "Three-Phase Tap Changer Transformer Pn MVA, Up / Us kV"/3(Tap position) -> Scope7/1  "Tap position"
  connections:
  Three-Phase V-I Measurement/LConn2 -- B/RConn1
  "Three-Phase Tap Changer Transformer Pn MVA, Up / Us kV"/LConn3 -- Three-Phase V-I Measurement/RConn3
  "Three-Phase Tap Changer Transformer Pn MVA, Up / Us kV"/RConn3 -- Three-Phase V-I Measurement1/LConn3
  "Three-Phase Tap Changer Transformer Pn MVA, Up / Us kV"/LConn1 -- Three-Phase V-I Measurement/RConn1
  "Three-Phase Tap Changer Transformer Pn MVA, Up / Us kV"/RConn2 -- Three-Phase V-I Measurement1/LConn2
  "Three-Phase Tap Changer Transformer Pn MVA, Up / Us kV"/LConn2 -- Three-Phase V-I Measurement/RConn2
  "Three-Phase Tap Changer Transformer Pn MVA, Up / Us kV"/RConn1 -- Three-Phase V-I Measurement1/LConn1
  Three-Phase V-I Measurement/LConn3 -- C/RConn1
  Three-Phase V-I Measurement1/RConn2 -- b/RConn1
  Three-Phase V-I Measurement/LConn1 -- A/RConn1
  Three-Phase V-I Measurement1/RConn3 -- c/RConn1
  Three-Phase V-I Measurement1/RConn1 -- a/RConn1

== system BenchmarkModel_Dynamic_TestCase/Subsystem1 ==
  f : Inport
  Controlled Voltage Source4 : powerlib/Electrical Sources/Controlled Voltage Source  Initialize=on  Source_Type=AC  Amplitude=20000*sqrt(2)/sqrt(3)  Phase=0  Frequency=50  Measurements=None
  Controlled Voltage Source5 : powerlib/Electrical Sources/Controlled Voltage Source  Initialize=on  Source_Type=AC  Amplitude=20000*sqrt(2)/sqrt(3)  Phase=120  Frequency=50  Measurements=None
  Controlled Voltage Source6 : powerlib/Electrical Sources/Controlled Voltage Source  Initialize=on  Source_Type=AC  Amplitude=20000*sqrt(2)/sqrt(3)  Phase=-120  Frequency=50  Measurements=None
  Ground2 : powerlib/Elements/Ground  LConnTagsString=a
  POWER CONVERTER1 : Subsystem
  Phase calculator1 : Subsystem
  A : PMIOPort  Side=Right
  B : PMIOPort  Port=2  Side=Right
  C : PMIOPort  Port=3  Side=Right
  wires:
  POWER CONVERTER1/1(Phase A) -> Controlled Voltage Source4/1
  Phase calculator1/1(phase) -> POWER CONVERTER1/1(phase3)
  POWER CONVERTER1/3(Phase C) -> Controlled Voltage Source5/1
  f/1 -> Phase calculator1/1(f1)
  POWER CONVERTER1/2(Phase B) -> Controlled Voltage Source6/1
  connections:
  Controlled Voltage Source6/RConn1 -- B/RConn1
  Controlled Voltage Source4/LConn1 -- Controlled Voltage Source5/LConn1 -- Controlled Voltage Source6/LConn1 -- Ground2/LConn1
  Controlled Voltage Source4/RConn1 -- A/RConn1
  Controlled Voltage Source5/RConn1 -- C/RConn1

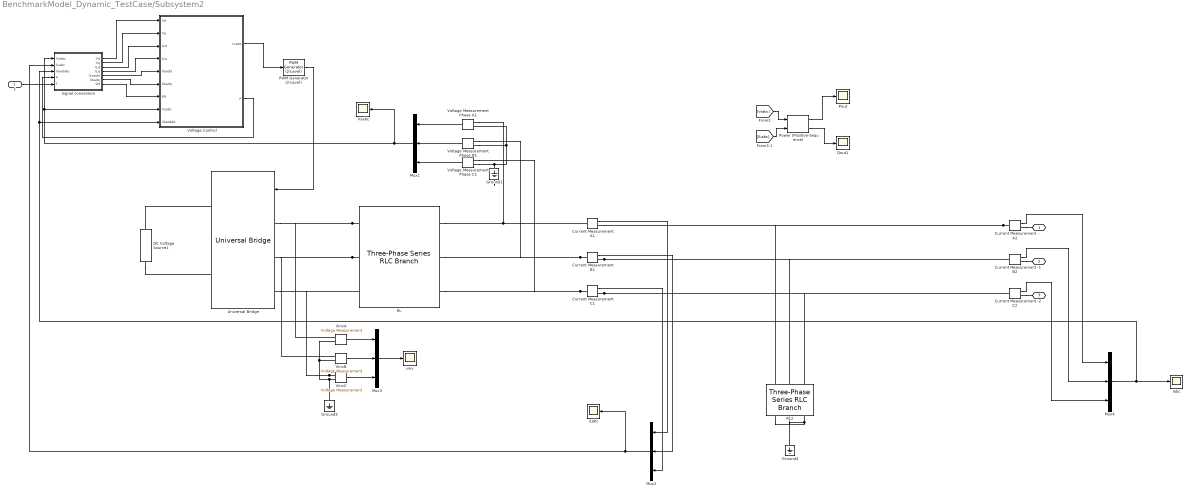
== system BenchmarkModel_Dynamic_TestCase/Subsystem2 ==
  f : Inport
  Current Measurement A1 : powerlib/Measurements/Current Measurement  PhasorSimulation=off  OutputType=Complex  PSBequivalent=0
  Current Measurement A2 : powerlib/Measurements/Current Measurement  PhasorSimulation=off  OutputType=Complex  PSBequivalent=0
  Current Measurement B1 : powerlib/Measurements/Current Measurement  PhasorSimulation=off  OutputType=Complex  PSBequivalent=0
  Current Measurement B2 : powerlib/Measurements/Current Measurement  PhasorSimulation=off  OutputType=Complex  PSBequivalent=0
  Current Measurement C1 : powerlib/Measurements/Current Measurement  PhasorSimulation=off  OutputType=Complex  PSBequivalent=0
  Current Measurement C2 : powerlib/Measurements/Current Measurement  PhasorSimulation=off  OutputType=Complex  PSBequivalent=0
  DC Voltage Source1 : powerlib/Electrical Sources/DC Voltage Source  Amplitude=800  Measurements=Voltage
  Ground1 : powerlib/Elements/Ground  LConnTagsString=a
  Ground3 : powerlib/Elements/Ground  LConnTagsString=a
  Ground4 : powerlib/Elements/Ground  LConnTagsString=a
  Mux{1..4} (4 alike) : Mux  Inputs=3
  PWM Generator (2-Level) : powerlib_meascontrol/Pulse & Signal Generators/PWM Generator (2-Level)  ModulatorType=Three-phase bridge (6 pulses)  ModulatorMode=Unsynchronized  Fc=16000  Pc=90  nF=27  MinMax="[ -1  1 ]"  SamplingTechnique=Natural  ModulatingSignals=off  m=0.8  Freq=60  Phase=0  Ts=5e-6  ShowCarrierOutport=off
  Pout : Scope
  Power (Positive-Sequence) : powerlib_meascontrol/Measurements/Power (Positive-Sequence)  Freq=50  Vinit=[1, 0]  Iinit=[1, 0]  Ts=1e-6
      settings: SourceProductBaseCode=PS
  Qout1 : Scope
  RL : powerlib/Elements/Three-Phase Series RLC Branch  LConnTagsString=A|B|C  RConnTagsString=A|B|C  BranchType=RL  Resistance=0.01  Inductance=0.01  Capacitance=1e-6  Measurements=Branch voltages and currents
  RL2 : powerlib/Elements/Three-Phase Series RLC Branch  LConnTagsString=A|B|C  RConnTagsString=A|B|C  BranchType=C  Resistance=0.001  Inductance=0.01  Capacitance=50e-6  Measurements=Branch voltages and currents
  Signal conversion : Subsystem
  Universal Bridge : powerlib/Power Electronics/Universal Bridge  Arms=3  SnubberResistance=1e5  SnubberCapacitance=inf  Device=Ideal Switches  Ron=1e-3  Lon=0  ForwardVoltages="[  0  0  ]"  ForwardVoltage=0  GTOparameters=[ 10e-6 , 20e-6 ]  IGBTparameters=[ 1e-6 , 2e-6 ]  Measurements=All voltages and currents  Measurements_2=None  converterType=Rectifier
  VinvA : powerlib/Measurements/Voltage Measurement  PhasorSimulation=off  OutputType=Complex  PSBequivalent=0
  VinvB : powerlib/Measurements/Voltage Measurement  PhasorSimulation=off  OutputType=Complex  PSBequivalent=0
  VinvC : powerlib/Measurements/Voltage Measurement  PhasorSimulation=off  OutputType=Complex  PSBequivalent=0
  Voltage Control : Subsystem
  Voltage Measurement Phase A1 : powerlib/Measurements/Voltage Measurement  PhasorSimulation=off  OutputType=Complex  PSBequivalent=0
  "Voltage Measurement Phase B1 " : powerlib/Measurements/Voltage Measurement  PhasorSimulation=off  OutputType=Complex  PSBequivalent=0
  "Voltage Measurement Phase C1 " : powerlib/Measurements/Voltage Measurement  PhasorSimulation=off  OutputType=Magnitude-Angle  PSBequivalent=0
  Vsabc : Scope
  iLabc : Scope
  iabc : Scope
  vinv : Scope
  - : PMIOPort  Side=Right
  -1 : PMIOPort  Port=2  Side=Right
  -2 : PMIOPort  Port=3  Side=Right
  wires:
  Mux1/1 -> Voltage Control/8(Vsabc), Signal conversion/1(Vsabc), Vsabc/1
  PWM Generator (2-Level)/1 -> Universal Bridge/1
  VinvA/1 -> Mux3/1
  Current Measurement C1/1 -> Mux2/3
  Voltage Measurement Phase A1/1 -> Mux1/1
  "Voltage Measurement Phase C1 "/1 -> Mux1/3
  Mux2/1 -> Signal conversion/2(ILabc), iLabc/1
  Power (Positive-Sequence)/1 -> Pout/1
  Current Measurement A1/1 -> Mux2/1
  Power (Positive-Sequence)/2 -> Qout1/1
  Current Measurement B1/1 -> Mux2/2
  [Vsabc] -> Power (Positive-Sequence)/1
  Voltage Control/1(mabc) -> PWM Generator (2-Level)/1
  VinvC/1 -> Mux3/3
  Mux3/1 -> vinv/1
  [ILabc] -> Power (Positive-Sequence)/2
  "Voltage Measurement Phase B1 "/1 -> Mux1/2
  VinvB/1 -> Mux3/2
  Mux4/1 -> iabc/1, Voltage Control/9(Iloadabc), Signal conversion/3(Iloadabc)
  Current Measurement A2/1 -> Mux4/1
  Current Measurement B2/1 -> Mux4/2
  Current Measurement C2/1 -> Mux4/3
  Signal conversion/4(ILq) -> Voltage Control/4(ILq)
  Signal conversion/3(ILd) -> Voltage Control/3(ILd)
  Signal conversion/5(ILoadd) -> Voltage Control/5(Iloadd)
  Signal conversion/2(Vq) -> Voltage Control/2(Vq)
  Signal conversion/6(Iloadq) -> Voltage Control/6(Iloadq)
  Signal conversion/1(Vd) -> Voltage Control/1(Vd)
  Signal conversion/7(Wt) -> Voltage Control/7(Wt)
  Voltage Control/2(P) -> Signal conversion/4(P)
  f/1 -> Signal conversion/5(f)
  connections:
  VinvC/LConn2 -- VinvB/LConn2 -- VinvA/LConn2 -- Ground3/LConn1
  Current Measurement C1/RConn1 -- RL2/LConn3 -- Current Measurement C2/LConn1
  RL/RConn1 -- Current Measurement A1/LConn1 -- Voltage Measurement Phase A1/LConn1
  "Voltage Measurement Phase B1 "/LConn2 -- "Voltage Measurement Phase C1 "/LConn2 -- Ground1/LConn1 -- Voltage Measurement Phase A1/LConn2
  RL2/RConn3 -- RL2/RConn1 -- Ground4/LConn1 -- RL2/RConn2
  Current Measurement A2/LConn1 -- Current Measurement A1/RConn1 -- RL2/LConn1
  RL/LConn1 -- Universal Bridge/LConn1 -- VinvA/LConn1
  Current Measurement B1/LConn1 -- RL/RConn2 -- "Voltage Measurement Phase B1 "/LConn1
  Current Measurement B1/RConn1 -- RL2/LConn2 -- Current Measurement B2/LConn1
  DC Voltage Source1/RConn1 -- Universal Bridge/RConn1
  Current Measurement C1/LConn1 -- RL/RConn3 -- "Voltage Measurement Phase C1 "/LConn1
  RL/LConn2 -- Universal Bridge/LConn2 -- VinvB/LConn1
  VinvC/LConn1 -- Universal Bridge/LConn3 -- RL/LConn3
  Current Measurement C2/RConn1 -- -2/RConn1
  DC Voltage Source1/LConn1 -- Universal Bridge/RConn2
  Current Measurement A2/RConn1 -- -/RConn1
  Current Measurement B2/RConn1 -- -1/RConn1

== system BenchmarkModel_Dynamic_TestCase/Synchronous Generator2 ==
  10 kW1 : powerlib/Elements/Three-Phase Parallel RLC Load  Commented=on  LConnTagsString=A|B|C  Configuration=Y (grounded)  NominalVoltage=400  Vabc=[1e3 1e3 1e3]  Vabcp=[1e3 1e3 1e3]  NominalFrequency=50  UnbalancedPower=off  ActivePower=10e3  InductivePower=0  CapacitivePower=0  Pabc=[10e3 9e3 11e3]  QLabc=[100 90 110]  QCabc=[100 90 110]  Pabcp=[10e3 9e3 11e3]  QLabcp=[100 90 110]  QCabcp=[100 90 110]  Measurements=None  LoadType=constant Z
  20 kW1 : powerlib/Elements/Three-Phase Parallel RLC Load  LConnTagsString=A|B|C  Configuration=Y (grounded)  NominalVoltage=400  Vabc=[1e3 1e3 1e3]  Vabcp=[1e3 1e3 1e3]  NominalFrequency=50  UnbalancedPower=off  ActivePower=5e3  InductivePower=0  CapacitivePower=0  Pabc=[10e3 9e3 11e3]  QLabc=[100 90 110]  QCabc=[100 90 110]  Pabcp=[10e3 9e3 11e3]  QLabcp=[100 90 110]  QCabcp=[100 90 110]  Measurements=None  LoadType=constant Z
  Bus Selector1 : BusSelector  OutputSignals="dq0 components.Stator voltage  vd (pu),dq0 components.Stator voltage  vq (pu),Mechanical.Rotor speed deviation  dw (pu),Output active power   Peo (pu),Mechanical.Rotor speed  wm  (pu)"
  Constant4 : Constant
  Constant5 : Constant  Value=0.358104
  Excitation System1 : sps_avr/Excitation System  tr=20e-3  reg=[ 300, 0.001 ]  exc=[ 1, 0 ]  tgr=[ 0, 0 ]  damp=[ 0.001, 0.1 ]  sat=[ 0, 0 ]  lim=[ -11.5, 11.5, 0 ]  v0=[1,1.19762]
      settings: SourceProductBaseCode=PS
  Iabc1 : Scope
  Potencia Pm1 : Scope
  Synchronous Machine Miain grid 60 kVA/400 V : powerlib/Machines/Synchronous Machine pu Standard  PresetModel=No  MechanicalLoad=Mechanical power Pm  ShowDetailedParameters=on  RotorType=Salient-pole  Units=per unit standard parameters  MeasurementBus=off  NominalParameters=[6e+04 400 50]  Reactances1=[ 1.81, 0.3, 0.23, 1.76, 0.65, 0.25, 0.15 ]  Reactances2=[2.24 0.17 0.12 1.02 0.13 0.08]  dAxisTimeConstants=Short-circuit  qAxisTimeConstants=Short-circuit  TimeConstants1="[ 4.4849  0.0681  0.1  ]"  TimeConstants2=[ 8.0, 0.03, 1.0, 0.07 ]  TimeConstants3="[  4.49  0.0681  0.0513  ]"  TimeConstants4=[ 8.0, 0.03, 0.3371, 0.0295 ]  TimeConstants5=[ 1.01, 0.053, 0.1 ]  TimeConstants6=[ 1.3201, 0.023, 1.0, 0.07 ]  TimeConstants7=[0.012 0.003 0.003]  TimeConstants8=[ 1.3201, 0.0231, 0.3371, 0.0295 ]  StatorResistance=0.037875  Mechanical=[0.1028 0.02056 2]  PolePairs=20  InitialConditions=[0 -71.4398 0.333336 0.333336 0.333336 0 -120 120 1.19762]  SetSaturation=on  Saturation=[0.6404,0.7127,0.8441,0.9214,0.9956,1.082,1.19,1.316,1.457;0.7,0.7698,0.8872,0.9466,0.9969,1.046,1.1,1.151,1.201]  LoadFlowParameters=[2 20000 0 0 0]  TsPowergui=0  TsBlock=-1  IterativeModel=Trapezoidal non iterative  IterativeDiscreteModel=Trapezoidal non iterative  BusType=PV  Pref=0  Qref=0  Qmin=-inf  Qmax=inf  PLF=0  QLF=0
  Terminator5 : Terminator
  Three-Phase V-I Measurement2 : powerlib/Measurements/Three-Phase V-I Measurement  VoltageMeasurement=phase-to-ground  SetLabelV=off  LabelV=Vabc  Vpu=off  VpuLL=off  CurrentMeasurement=yes  SetLabelI=off  LabelI=Iabc  Ipu=off  Pbase=100e6  Vbase=500e3  OutputType=Complex  PhasorSimulation=on  PSBequivalent=0
  Three-Phase Breaker3 : powerlib/Elements/Three-Phase Breaker  InitialState=open  SwitchA=on  SwitchB=on  SwitchC=on  SwitchTimes=0.25  External=off  BreakerResistance=0.01  SnubberResistance=1e6  SnubberCapacitance=inf  Measurements=None
  Vabc1 : Scope
  Vrotor Pm1 : Scope
  a : PMIOPort  Side=Right
  b : PMIOPort  Port=2  Side=Right
  c : PMIOPort  Port=3  Side=Right
  wires:
  Bus Selector1/4 -> Potencia Pm1/1  "<Output active power   Peo (pu)>"
  Excitation System1/1 -> Synchronous Machine Miain grid 60 kVA/400 V/2
  Three-Phase V-I Measurement2/1 -> Vabc1/1
  Synchronous Machine Miain grid 60 kVA/400 V/1 -> Bus Selector1/1
  Bus Selector1/5 -> Vrotor Pm1/1  "<Rotor speed  wm  (pu)>"
  Bus Selector1/3 -> Excitation System1/4  "<Rotor speed deviation  dw (pu)>"
  Constant4/1 -> Excitation System1/1
  Three-Phase V-I Measurement2/2 -> Iabc1/1
  Bus Selector1/1 -> Excitation System1/3  "<Stator voltage  vd (pu)>"
  Bus Selector1/2 -> Excitation System1/2  "<Stator voltage  vq (pu)>"
  Constant5/1 -> Synchronous Machine Miain grid 60 kVA/400 V/1
  connections:
  Three-Phase Breaker3/RConn2 -- b/RConn1 -- 10 kW1/LConn2
  20 kW1/LConn1 -- Three-Phase V-I Measurement2/RConn1 -- Three-Phase Breaker3/LConn1
  Three-Phase Breaker3/LConn3 -- Three-Phase V-I Measurement2/RConn3 -- 20 kW1/LConn3
  Three-Phase Breaker3/RConn1 -- a/RConn1 -- 10 kW1/LConn1
  Three-Phase Breaker3/RConn3 -- c/RConn1 -- 10 kW1/LConn3
  Three-Phase Breaker3/LConn2 -- Three-Phase V-I Measurement2/RConn2 -- 20 kW1/LConn2
  Synchronous Machine Miain grid 60 kVA/400 V/RConn1 -- Three-Phase V-I Measurement2/LConn1
  Synchronous Machine Miain grid 60 kVA/400 V/RConn3 -- Three-Phase V-I Measurement2/LConn3
  Synchronous Machine Miain grid 60 kVA/400 V/RConn2 -- Three-Phase V-I Measurement2/LConn2
